simulink model "ParabolicTrough"  (R2025a)
settings: Solver=ode45  StartTime=0.0  StopTime=2000  RelTol=1e-3
undefined symbols (not defined in the file): C, ccp, Gsun
libraries: slpidlib x1
settings Model: Creator=charizardmigo  LastModifiedBy=charizardmigo

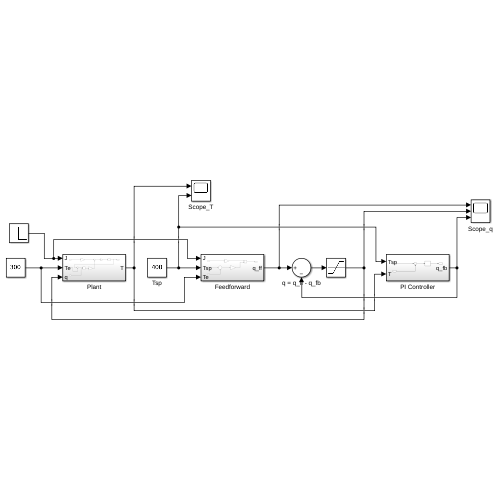
[thumbnail: Simulink's stored preview of the top-level diagram]
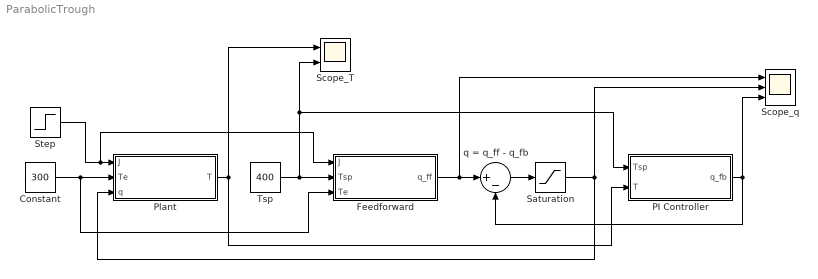
== system ParabolicTrough ==
  Constant : Constant  Value=300
  Feedforward : Subsystem
  PI Controller : Subsystem
  Plant : Subsystem
  Saturation : Saturate  UpperLimit=10  LowerLimit=0
  Scope_T : Scope  NumInputPorts=2
      settings: ActiveDisplayYMinimum=399.00374807364017  ActiveDisplayYMaximum=401.68501743527361
  Scope_q : Scope  NumInputPorts=3
      settings: ActiveDisplayYMinimum=2.4381528265739218  ActiveDisplayYMaximum=6.9643873110791414
  Step : Step  Time=500  Before=0.8  After=0.6  SampleTime=0
  Tsp : Constant  Value=400
  q = q_ff - q_fb : Sum  Inputs=|+-
  wires:
  Step/1 -> Plant/1(J), Feedforward/1(J)
  Plant/1(T) -> PI Controller/2(T), Scope_T/1
  Feedforward/1(q_ff) -> q = q_ff - q_fb/1, Scope_q/1
  q = q_ff - q_fb/1 -> Saturation/1
  Saturation/1 -> Scope_q/2, Plant/3(q)
  Tsp/1 -> PI Controller/1(Tsp), Scope_T/2, Feedforward/2(Tsp)
  PI Controller/1(q_fb) -> Scope_q/3, q = q_ff - q_fb/2
  Constant/1 -> Feedforward/3(Te), Plant/2(Te)

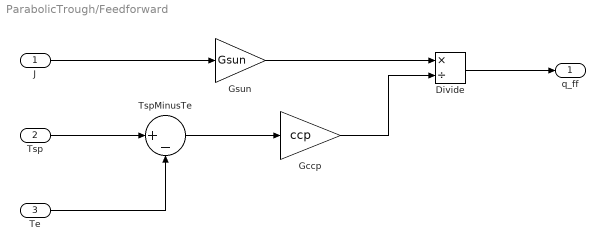
== system ParabolicTrough/Feedforward ==
  J : Inport
  Tsp : Inport  Port=2
  Te : Inport  Port=3
  Divide : Product  Inputs=*/
  Gccp : Gain  Gain=ccp
  Gsun : Gain  Gain=Gsun
  TspMinusTe : Sum  Inputs=|+-
  q_ff : Outport
  wires:
  J/1 -> Gsun/1
  Divide/1 -> q_ff/1
  Tsp/1 -> TspMinusTe/1
  Te/1 -> TspMinusTe/2
  Gsun/1 -> Divide/1
  TspMinusTe/1 -> Gccp/1
  Gccp/1 -> Divide/2

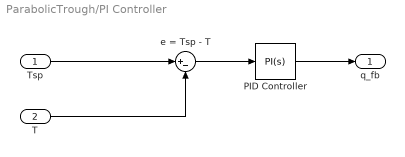
== system ParabolicTrough/PI Controller ==
  Tsp : Inport
  T : Inport  Port=2
  PID Controller : slpidlib/PID Controller  Controller=PI  Form=Parallel  TimeDomain=Continuous-time  UseExternalTs=off  SampleTime=-1  IntegratorMethod=Forward Euler  FilterMethod=Forward Euler  ControllerParametersSource=internal  P=0.165  I=0.014  UseKiTs=off  D=0  UseExternalDerivativeSource=off  N=100  UseFilter=on  TunerSelectOption=Transfer Function Based (PID Tuner App)  InitialConditionSource=internal  InitialConditionForIntegrator=0  InitialConditionForFilter=0  DifferentiatorICPrevScaledInput=0  ExternalReset=none  TrackingMode=off  Kt=1  LimitOutput=off  SatLimitsSource=internal  UpperSaturationLimit=inf  LowerSaturationLimit=-inf  LinearizeAsGain=on  AntiWindupMode=none  Kb=1  LimitIntegrator=off  UpperIntegratorSaturationLimit=inf  LowerIntegratorSaturationLimit=-inf  POutMin=[]  POutMax=[]  IOutMin=[]  IOutMax=[]  DOutMin=[]  DOutMax=[]  NOutMin=[]  NOutMax=[]  SumOutMin=[]  SumOutMax=[]  SaturationOutMin=[]  SaturationOutMax=[]  PParamMin=[]  PParamMax=[]  IParamMin=[]  IParamMax=[]  DParamMin=[]  DParamMax=[]  NParamMin=[]  NParamMax=[]  KbParamMin=[]  KbParamMax=[]  KtParamMin=[]  KtParamMax=[]  KbOutMin=[]  KbOutMax=[]  KtOutMin=[]  KtOutMax=[]  IntegratorOutMin=[]  IntegratorOutMax=[]  FilterOutMin=[]  FilterOutMax=[]  SumI1OutMin=[]  SumI1OutMax=[]  SumI2OutMin=[]  SumI2OutMax=[]  SumI3OutMin=[]  SumI3OutMax=[]  SumI4OutMin=[]  SumI4OutMax=[]  SumDOutMin=[]  SumDOutMax=[]  DifferentiatorOutMin=[]  DifferentiatorOutMax=[]  FilterDiffOutCoefMin=[]  FilterDiffOutCoefMax=[]  ReciprocalOutMin=[]  ReciprocalOutMax=[]  SumDenOutMin=[]  SumDenOutMax=[]  SumNumOutMin=[]  SumNumOutMax=[]  DivideOutMin=[]  DivideOutMax=[]  UdiffTsProdOutMin=[]  UdiffTsProdOutMax=[]  NTsProdOutMin=[]  NTsProdOutMax=[]  UintegralTsProdOutMin=[]  UintegralTsProdOutMax=[]  UngainTsProdOutMin=[]  UngainTsProdOutMax=[]  ClampingZeroOutDataTypeStr=Inherit: Inherit via back propagation  ClampingZeroOutMin=[]  ClampingZeroOutMax=[]  FilterDenConstantOutDataTypeStr=Inherit: Inherit via back propagation  FilterDenConstantOutMin=[]  FilterDenConstantOutMax=[]  PCopyOutDataTypeStr=Inherit: Inherit via back propagation  PCopyOutMin=[]  PCopyOutMax=[]  NCopyOutDataTypeStr=Inherit: Inherit via back propagation  NCopyOutMin=[]  NCopyOutMax=[]  IntegratorContinuousStateAttributes=''  IntegratorStateMustResolveToSignalObject=off  IntegratorRTWStateStorageClass=Auto  FilterContinuousStateAttributes=''  FilterStateMustResolveToSignalObject=off  FilterRTWStateStorageClass=Auto  ParallelPVariant=InternalParameters  IdealPVariant=Disabled  IVariant=InternalParameters  DVariant=Disabled  IntegratorVariant=Continuous  SatVariant=Disabled  AWVariant=Passthrough  PCopyVariant=Disabled  TRVariant=Disabled  FdbkBlocksVariant=Forward  IdealPFdbkVariant=Disabled  SatFdbkVariant=Disabled  DerivativeFilterVariant=Disabled  NVariant=Disabled  NCopyVariant=Disabled_SignalSpec  FilterICVariant=Disabled  IntegratorICVariant=InternalICs  ExternalResetVariant=Disabled  TRSumVariant=Passthrough  SumFdbkVariant=Disabled  SumVariant=Sum_PI  TsampFilterVariant=InternalTs  TsampNgainVariant=Passthrough  TsampIntegralVariant=Disabled_SignalSpec  ExternalSaturationOutDataTypeStr=Inherit: Same as second input  DerivativeSourceVariant=Disabled  PreIntVariant=InternalPreInt
  e = Tsp - T : Sum  Inputs=|+-
  q_fb : Outport
  wires:
  T/1 -> e = Tsp - T/2
  Tsp/1 -> e = Tsp - T/1
  e = Tsp - T/1 -> PID Controller/1
  PID Controller/1 -> q_fb/1

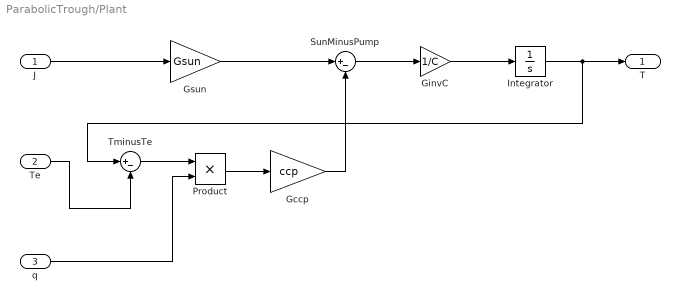
== system ParabolicTrough/Plant ==
  J : Inport
  Te : Inport  Port=2
  q : Inport  Port=3
  Gccp : Gain  Gain=ccp
  GinvC : Gain  Gain=1/C
  Gsun : Gain  Gain=Gsun
  Integrator : Integrator  InitialCondition=400
  Product : Product
  SunMinusPump : Sum  Inputs=|+-
  TminusTe : Sum  Inputs=|+-
  T : Outport
  wires:
  J/1 -> Gsun/1
  Integrator/1 -> T/1, TminusTe/1
  Te/1 -> TminusTe/2
  SunMinusPump/1 -> GinvC/1
  GinvC/1 -> Integrator/1
  TminusTe/1 -> Product/1
  q/1 -> Product/2
  Product/1 -> Gccp/1
  Gccp/1 -> SunMinusPump/2
  Gsun/1 -> SunMinusPump/1
